simulink model "io308"  (Simulink 6.0)
settings: Solver=FixedStepDiscrete  StartTime=0.0  StopTime=300  RelTol=1e-3
PreLoadFcn:
  | setxpcenv('CAN','PC104');updatexpcenv(1);
undefined symbols (not defined in the file or in its folder): bit, Standard
libraries: xpclib x3
CloseFcn:
  | setxpcenv('CAN','None');updatexpcenv(1)
settings Model: Creator=mvetsch  LastModifiedBy=ekbas  ExtModeArmWhenConnect=off  BufferReuse=off
settings DataIOCC: SaveFormat=Structure  SignalLoggingName=sigsOut
settings OptimizationCC: BlockReduction=off  BooleanDataType=off  InlineInvariantSignals=off  OptimizeBlockIOStorage=off  BufferReuse=off  LocalBlockOutputs=off
settings DebuggingCC: CheckExecutionContextPreStartOutputMsg=on  CheckExecutionContextRuntimeOutputMsg=on  SolverPrmCheckMsg=none
settings HardwareCC: TargetUnknown=on
settings RTWCC: SystemTargetFile=xpctarget.tlc  TemplateMakefile=xpc_default_tmf  ProcessScript=xpctarget_make_rtw_hook
settings xpcTargetCC: TargetFcnLib=ansi_tfl_tmw.mat  GenFloatMathFcnCalls=ANSI_C
settings SFSimCC: SFSimApplyToAllLibs=on  SFSimBuildMode=Incremental

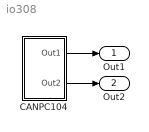
== system io308 ==
  CANPC104 : Subsystem  PropExecContextAcrossSSBoundary=on
  Out1 : Outport
  Out2 : Outport  Port=2
  wires:
  CANPC104/1(Out1) -> Out1/1
  CANPC104/2(Out2) -> Out2/1

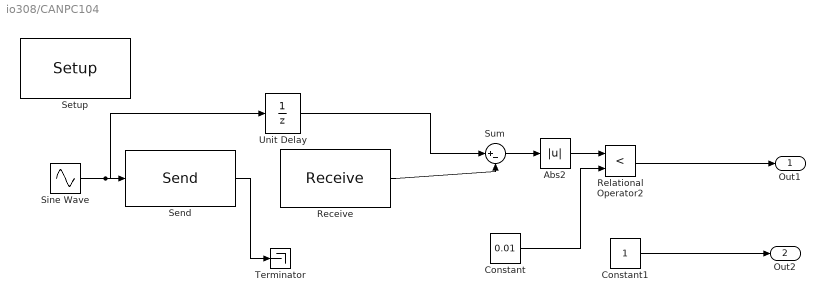
== system io308/CANPC104 ==
  Abs2 : Abs  SaturateOnIntegerOverflow=on
  Constant : Constant  Value=0.01
  Constant1 : Constant
  "Receive " : xpclib/CAN/Softing/CAN-AC2-104 SJA 1000/Receive   board=1  canPort=CAN 2  range=Standard (11-bit)  ids=[50]  output=Data  inten=off  ts=0.01  ididx=[0]
  Relational Operator2 : RelationalOperator  Operator=<
  "Send " : xpclib/CAN/Softing/CAN-AC2-104 SJA 1000/Send   board=1  canPort=CAN 1  range=Standard (11-bit)  ids=[50]  sizes=[8]  output=on  ts=0.01  ididx=[0]
  "Setup " : xpclib/CAN/Softing/CAN-AC2-104 SJA 1000/Setup   board=1  can1Baudrate=1 MBaud  can1UserBR=[1,1,4,3]  can2Baudrate=1 MBaud  can2UserBR=[1,1,4,3]  init=[]  term=[]  ioBaseAddressL=0x300  memBaseAddressL=0xd0000  intNo=None
  Sine Wave : Sin  Frequency=5  SampleTime=0.01
  Sum : Sum  Inputs=|+-  SaturateOnIntegerOverflow=on
  Terminator : Terminator
  Unit Delay : UnitDelay  SampleTime=-1
  Out1 : Outport
  Out2 : Outport  Port=2
  wires:
  Sine Wave/1 -> "Send "/1, Unit Delay/1
  "Receive "/1 -> Sum/2
  Sum/1 -> Abs2/1
  Abs2/1 -> Relational Operator2/1
  Relational Operator2/1 -> Out1/1
  Constant/1 -> Relational Operator2/2
  Unit Delay/1 -> Sum/1
  "Send "/1 -> Terminator/1
  Constant1/1 -> Out2/1
